simulink model "yaduraj_mli_231040124"  (R2023a)
settings: Solver=ode3  StartTime=0.0  StopTime=.05  RelTol=1e-3  EnableMultiTasking=on
InitFcn:
  | Fs=1550;
  | Ts=1/1550;
libraries: simulink x42, spsIGBTDiodeLib x36, spsDCVoltageSourceLib x9, spsVoltageMeasurementLib x9, spsSeriesRLCBranchLib x3, spsGroundLib x2, sps_lib x1
settings Model: Creator=yadur  LastModifiedBy=yadur
settings SolverCC: AlgebraicLoopSolver=TrustRegion  AutoInsertRateTranBlk=on
settings DataIOCC: SaveFormat=StructureWithTime  ReturnWorkspaceOutputs=off
settings DebuggingCC: ArithmeticOperatorsInVariantConditions=warning
settings SFSimCC: CustomCodeUndefinedFunction=UseInterfaceOnly

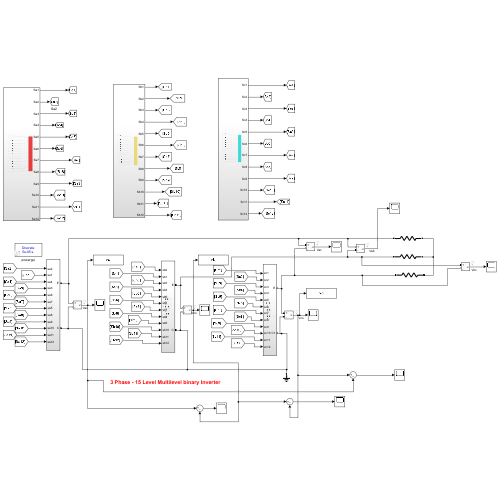
[thumbnail: Simulink's stored preview of the top-level diagram]
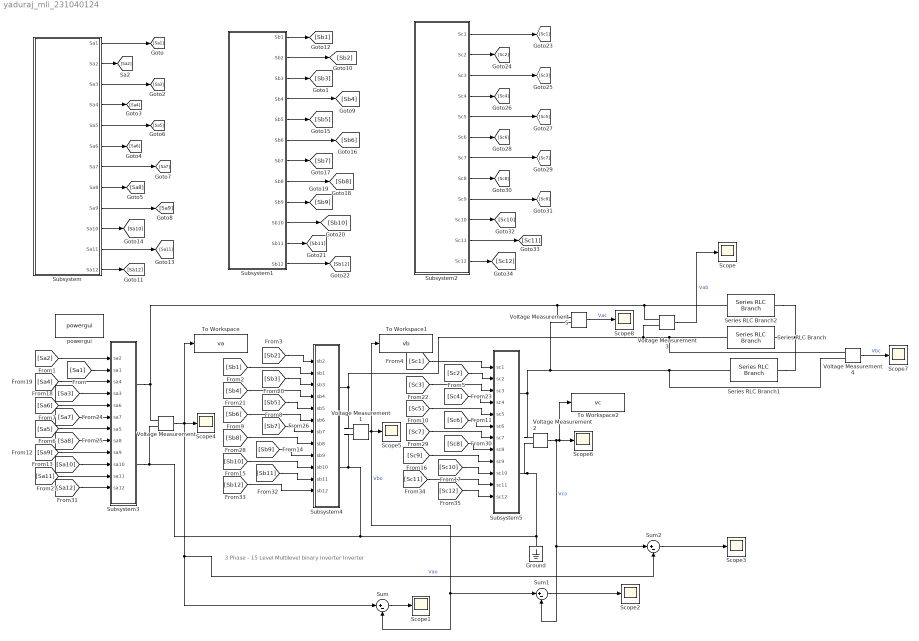
== system yaduraj_mli_231040124 ==
  note: 3 Phase - 15 Level Multilevel binary Inverter Inverter
  Ground : spsGroundLib/Ground  LConnTagsString=a
  Scope{,1..8} (9 alike) : Scope
  Series RLC Branch : spsSeriesRLCBranchLib/Series RLC Branch  LConnTagsString=__new0  RConnTagsString=__new0  BranchType=R  Resistance=1  Inductance=1e-3  SetiL0=off  InitialCurrent=0  Capacitance=1e-6  Setx0=off  InitialVoltage=0  Measurements=None
  Series RLC Branch1 : spsSeriesRLCBranchLib/Series RLC Branch  LConnTagsString=__new0  RConnTagsString=__new0  BranchType=R  Resistance=1  Inductance=1e-3  SetiL0=off  InitialCurrent=0  Capacitance=1e-6  Setx0=off  InitialVoltage=0  Measurements=None
  Series RLC Branch2 : spsSeriesRLCBranchLib/Series RLC Branch  LConnTagsString=__new0  RConnTagsString=__new0  BranchType=R  Resistance=1  Inductance=1e-3  SetiL0=off  InitialCurrent=0  Capacitance=1e-6  Setx0=off  InitialVoltage=0  Measurements=None
  Subsystem : Subsystem
  Subsystem1 : Subsystem
  Subsystem2 : Subsystem
  Subsystem3 : Subsystem
  Subsystem4 : Subsystem
  Subsystem5 : Subsystem
  Sum : Sum  Inputs=|+-
  Sum1 : Sum  Inputs=|+-
  Sum2 : Sum  Inputs=|+-
  To Workspace : ToWorkspace  VariableName=va  SampleTime=-1
      settings: Save2DSignal=2-D array (concatenate along first dimension)
  To Workspace1 : ToWorkspace  VariableName=vb  SampleTime=-1
      settings: Save2DSignal=2-D array (concatenate along first dimension)
  To Workspace2 : ToWorkspace  VariableName=vc  SampleTime=-1
      settings: Save2DSignal=2-D array (concatenate along first dimension)
  Voltage Measurement{,1..5} (6 alike) : spsVoltageMeasurementLib/Voltage Measurement  PhasorSimulation=off  OutputType=Complex  PSBequivalent=0
  powergui : sps_lib/powergui  Priority=1  SimulationMode=Discrete  SampleTime=50e-6  frequency=60  Iterations=50  frequencyindice=0  Pbase=100e6  ErrMax=1e-4  UnitsV=kV  UnitsW=MW  buscounter=0  FunctionMessages=off  echomessages=off  EnableUseOfTLC=off  CurrentSourceSwitches=off  DisableSnubberDevices=off  DisableRonSwitches=off  DisableVfSwitches=off  DisplayEquations=off  AutomaticDiscreteSolvers=off  SolverType=Tustin/Backward Euler (TBE)  Interpol=off  ExternalGateDelay=off  methode=off  Ts=100  x0status=blocks  SPID=on  SwTol=0  HookPort=off  NonlinearTolerance=1e-4  nMaxIteration=100  ContinueOnMaxIteration=off  RestoreLinks=warning  ResistiveCurrentMeasurement=off  Frange=[0:2:500]  Ylog=off  Xlog=on  ShowGrid=off  save=off  variable=ZData  structure=0  ZoomFFT=off  StartTime=0.0  cycles=1  DisplayStyle=1  fundamental=60  FreqAxis=off  MaxFrequency=1000  frequencyindicesteady=1  RmsSteady=1  display=off
  wires:
  Subsystem2/2(Sc2) -> [Sc2]
  Subsystem2/1(Sc1) -> [Sc1]
  Subsystem2/7(Sc7) -> [Sc7]
  Subsystem2/6(Sc6) -> [Sc6]
  Subsystem2/4(Sc4) -> [Sc4]
  Subsystem2/3(Sc3) -> [Sc3]
  Subsystem2/5(Sc5) -> [Sc5]
  [Sc11] -> Subsystem5/11(sc11)
  [Sc6] -> Subsystem5/6(sc6)
  [Sc8] -> Subsystem5/8(sc8)
  [Sc7] -> Subsystem5/7(sc7)
  [Sc10] -> Subsystem5/10(sc10)
  [Sc9] -> Subsystem5/9(sc9)
  Subsystem2/8(Sc8) -> [Sc8]
  [Sc5] -> Subsystem5/5(sc5)
  [Sc4] -> Subsystem5/4(sc4)
  [Sc1] -> Subsystem5/1(sc1)
  Subsystem1/12(Sb12) -> [Sb12]
  Subsystem1/9(Sb9) -> [Sb9]
  [Sc12] -> Subsystem5/12(sc12)
  Subsystem1/6(Sb6) -> [Sb6]
  Subsystem1/11(Sb11) -> [Sb11]
  Subsystem1/5(Sb5) -> [Sb5]
  Subsystem1/8(Sb8) -> [Sb8]
  Subsystem1/7(Sb7) -> [Sb7]
  Subsystem1/2(Sb2) -> [Sb2]
  Subsystem1/4(Sb4) -> [Sb4]
  Subsystem1/3(Sb3) -> [Sb3]
  Subsystem1/1(Sb1) -> [Sb1]
  [Sc2] -> Subsystem5/2(sc2)
  Subsystem/4(Sa4) -> [Sa4]
  Subsystem/10(Sa10) -> [Sa10]
  Subsystem/9(Sa9) -> [Sa9]
  Subsystem/11(Sa11) -> [Sa11]
  [Sa12] -> Subsystem3/12(sa12)
  [Sa9] -> Subsystem3/9(sa9)
  [Sa8] -> Subsystem3/8(sa8)
  [Sa5] -> Subsystem3/7(sa5)
  [Sa6] -> Subsystem3/5(sa6)
  [Sa4] -> Subsystem3/3(sa4)
  [Sa1] -> Subsystem3/2(sa1)
  [Sa2] -> Subsystem3/1(sa2)
  Subsystem/6(Sa6) -> [Sa6]
  [Sa3] -> Subsystem3/4(sa3)
  Subsystem/5(Sa5) -> [Sa5]
  [Sa10] -> Subsystem3/10(sa10)
  Subsystem/1(Sa1) -> [Sa1]
  Subsystem/7(Sa7) -> [Sa7]
  Subsystem1/10(Sb10) -> [Sb10]
  [Sc3] -> Subsystem5/3(sc3)
  Subsystem2/12(Sc12) -> [Sc12]
  Subsystem2/10(Sc10) -> [Sc10]
  Subsystem2/11(Sc11) -> [Sc11]
  [Sa11] -> Subsystem3/11(sa11)
  Subsystem2/9(Sc9) -> [Sc9]
  Subsystem/8(Sa8) -> [Sa8]
  Subsystem/3(Sa3) -> [Sa3]
  Subsystem/12(Sa12) -> [Sa12]
  [Sb12] -> Subsystem4/12(sb12)
  [Sb11] -> Subsystem4/11(sb11)
  [Sb9] -> Subsystem4/9(sb9)
  [Sb10] -> Subsystem4/10(sb10)
  [Sb8] -> Subsystem4/8(sb8)
  Subsystem/2(Sa2) -> [Sa2]
  [Sb7] -> Subsystem4/7(sb7)
  [Sb6] -> Subsystem4/6(sb6)
  [Sb3] -> Subsystem4/3(sb3)
  [Sb2] -> Subsystem4/1(sb2)
  [Sb1] -> Subsystem4/2(sb1)
  [Sa7] -> Subsystem3/6(sa7)
  [Sb5] -> Subsystem4/5(sb5)
  [Sb4] -> Subsystem4/4(sb4)
  Voltage Measurement3/1 -> Scope/1  "Vab"
  Voltage Measurement/1 -> Scope4/1, Sum2/2, Sum/1, To Workspace/1  "Vao"
  Voltage Measurement1/1 -> To Workspace1/1, Scope5/1, Sum1/1, Sum/2  "Vbo"
  Sum/1 -> Scope1/1
  Voltage Measurement2/1 -> Scope6/1, To Workspace2/1, Sum2/1, Sum1/2  "Vco"
  Sum1/1 -> Scope2/1
  Sum2/1 -> Scope3/1
  Voltage Measurement4/1 -> Scope7/1  "Vbc"
  Voltage Measurement5/1 -> Scope8/1  "Vac"
  connections:
  Subsystem5/RConn2 -- Voltage Measurement1/LConn2 -- Subsystem4/RConn2 -- Voltage Measurement/LConn2 -- Subsystem3/RConn2 -- Ground/LConn1 -- Voltage Measurement2/LConn2
  Subsystem4/RConn1 -- Voltage Measurement3/LConn2 -- Voltage Measurement4/LConn1 -- Series RLC Branch/LConn1 -- Voltage Measurement1/LConn1
  Subsystem3/RConn1 -- Voltage Measurement5/LConn1 -- Voltage Measurement3/LConn1 -- Series RLC Branch2/LConn1 -- Voltage Measurement/LConn1
  Subsystem5/RConn1 -- Voltage Measurement5/LConn2 -- Voltage Measurement4/LConn2 -- Series RLC Branch1/LConn1 -- Voltage Measurement2/LConn1
  Series RLC Branch1/RConn1 -- Series RLC Branch2/RConn1 -- Series RLC Branch/RConn1

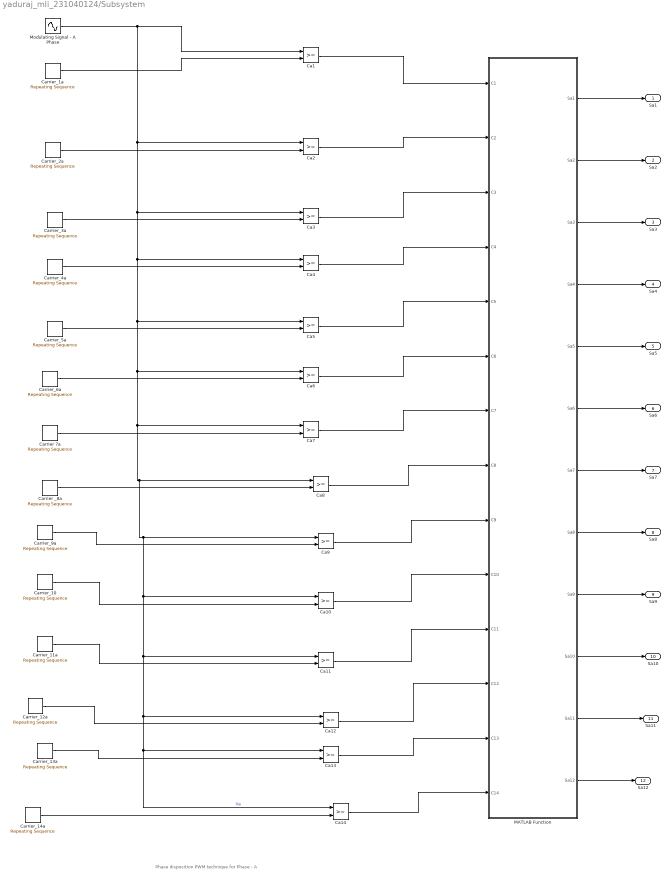
== system yaduraj_mli_231040124/Subsystem ==
  note: Phase disposition PWM technique for Phase - A
  Ca{1..14} (14 alike) : RelationalOperator  OutDataTypeStr=boolean  RndMeth=Simplest  InputSameDT=off
  Carrier 7a : simulink/Sources/Repeating Sequence  rep_seq_t="[0  1/2 1]*Ts"  rep_seq_y="[0 2/14  0]"
  Carrier _8a : simulink/Sources/Repeating Sequence  rep_seq_t="[0  1/2 1]*Ts"  rep_seq_y="[-2/14 0  -2/14  ]"
  Carrier_10 : simulink/Sources/Repeating Sequence  rep_seq_t="[0  1/2 1]*Ts"  rep_seq_y="[-6/14 -4/14  -6/14]"
  Carrier_11a : simulink/Sources/Repeating Sequence  rep_seq_t="[0  1/2 1]*Ts"  rep_seq_y="[-8/14 -6/14  -8/14]"
  Carrier_12a : simulink/Sources/Repeating Sequence  rep_seq_t="[0  1/2 1]*Ts"  rep_seq_y="[-10/14 -8/14  -10/14]"
  Carrier_13a : simulink/Sources/Repeating Sequence  rep_seq_t="[0  1/2 1]*Ts"  rep_seq_y="[-12/14 -10/14  -12/14]"
  Carrier_14a : simulink/Sources/Repeating Sequence  rep_seq_t="[0  1/2 1]*Ts"  rep_seq_y="[-14/14 -12/14  -14/14]"
  Carrier_1a : simulink/Sources/Repeating Sequence  rep_seq_t="[0  1/2 1]*Ts"  rep_seq_y="[12/14 14/14  12/14]"
  Carrier_2a : simulink/Sources/Repeating Sequence  rep_seq_t="[0  1/2 1]*Ts"  rep_seq_y="[10/14 12/14  10/14]"
  Carrier_3a : simulink/Sources/Repeating Sequence  rep_seq_t="[0  1/2 1]*Ts"  rep_seq_y="[8/14 10/14  8/14]"
  Carrier_4a : simulink/Sources/Repeating Sequence  rep_seq_t="[0  1/2 1]*Ts"  rep_seq_y="[6/14 8/14  6/14]"
  Carrier_5a : simulink/Sources/Repeating Sequence  rep_seq_t="[0  1/2 1]*Ts"  rep_seq_y="[4/14 6/14  4/14]"
  Carrier_6a : simulink/Sources/Repeating Sequence  rep_seq_t="[0  1/2 1]*Ts"  rep_seq_y="[2/14 4/14  2/14]"
  Carrier_9a : simulink/Sources/Repeating Sequence  rep_seq_t="[0  1/2 1]*Ts"  rep_seq_y="[-4/14 -2/14  -4/14]"
  MATLAB Function : MATLAB Function  TreatAsAtomicUnit=on
  Modulating Signal - A Phase : Sin  Frequency=2*pi*50  SampleTime=1e-6
  Sa1 : Outport
  Sa2 : Outport  Port=2
  Sa3 : Outport  Port=3
  Sa4 : Outport  Port=4
  Sa5 : Outport  Port=5
  Sa6 : Outport  Port=6
  Sa7 : Outport  Port=7
  Sa8 : Outport  Port=8
  Sa9 : Outport  Port=9
  Sa10 : Outport  Port=10
  Sa11 : Outport  Port=11
  Sa12 : Outport  Port=12
  wires:
  Carrier _8a/1 -> Ca8/2
  Ca8/1 -> MATLAB Function/8(C8)
  Carrier_4a/1 -> Ca4/2
  Ca2/1 -> MATLAB Function/2(C2)
  Carrier_2a/1 -> Ca2/2
  Carrier_9a/1 -> Ca9/2
  Ca3/1 -> MATLAB Function/3(C3)
  MATLAB Function/8(Sa8) -> Sa8/1
  Modulating Signal - A Phase/1 -> Ca14/1, Ca13/1, Ca12/1, Ca11/1, Ca10/1, Ca9/1, Ca8/1, Ca7/1, Ca6/1, Ca5/1, Ca4/1, Ca3/1, Ca2/1, Ca1/1  "Va"
  Carrier_11a/1 -> Ca11/2
  Carrier_3a/1 -> Ca3/2
  Ca5/1 -> MATLAB Function/5(C5)
  MATLAB Function/1(Sa1) -> Sa1/1
  MATLAB Function/4(Sa4) -> Sa4/1
  Carrier_1a/1 -> Ca1/2
  Ca9/1 -> MATLAB Function/9(C9)
  Carrier_5a/1 -> Ca5/2
  MATLAB Function/5(Sa5) -> Sa5/1
  MATLAB Function/9(Sa9) -> Sa9/1
  Ca4/1 -> MATLAB Function/4(C4)
  Ca12/1 -> MATLAB Function/12(C12)
  MATLAB Function/6(Sa6) -> Sa6/1
  Carrier_6a/1 -> Ca6/2
  Ca1/1 -> MATLAB Function/1(C1)
  Ca13/1 -> MATLAB Function/13(C13)
  Ca14/1 -> MATLAB Function/14(C14)
  Ca6/1 -> MATLAB Function/6(C6)
  Carrier_12a/1 -> Ca12/2
  MATLAB Function/3(Sa3) -> Sa3/1
  Carrier_14a/1 -> Ca14/2
  MATLAB Function/10(Sa10) -> Sa10/1
  Ca10/1 -> MATLAB Function/10(C10)
  Carrier 7a/1 -> Ca7/2
  MATLAB Function/12(Sa12) -> Sa12/1
  MATLAB Function/7(Sa7) -> Sa7/1
  Carrier_10/1 -> Ca10/2
  Ca7/1 -> MATLAB Function/7(C7)
  Carrier_13a/1 -> Ca13/2
  MATLAB Function/2(Sa2) -> Sa2/1
  Ca11/1 -> MATLAB Function/11(C11)
  MATLAB Function/11(Sa11) -> Sa11/1

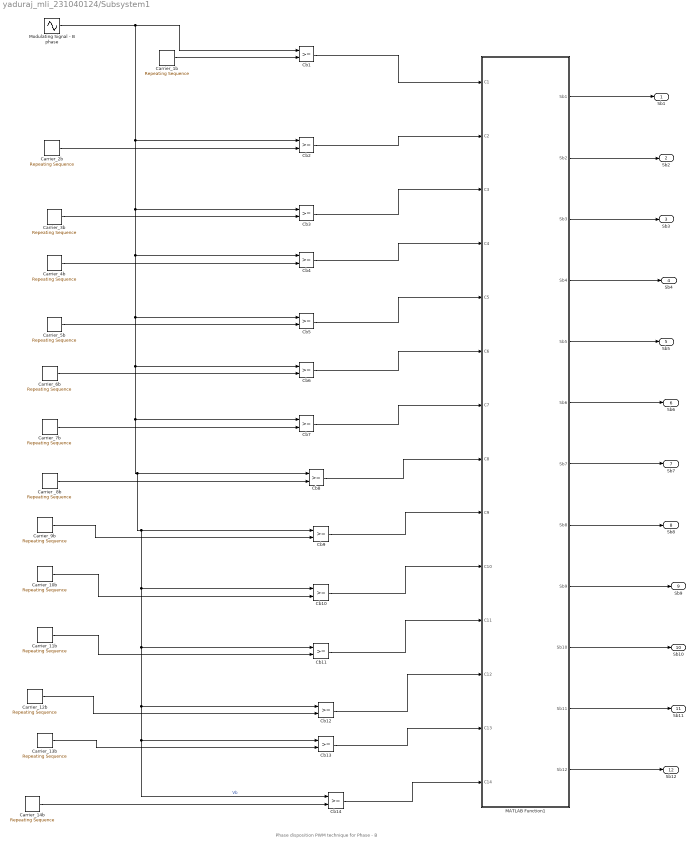
== system yaduraj_mli_231040124/Subsystem1 ==
  note: Phase disposition PWM technique for Phase - B
  Carrier _8b : simulink/Sources/Repeating Sequence  rep_seq_t="[0  1/2 1]*Ts"  rep_seq_y="[-2/14 0  -2/14  ]"
  Carrier_10b : simulink/Sources/Repeating Sequence  rep_seq_t="[0  1/2 1]*Ts"  rep_seq_y="[-6/14 -4/14  -6/14]"
  Carrier_11b : simulink/Sources/Repeating Sequence  rep_seq_t="[0  1/2 1]*Ts"  rep_seq_y="[-8/14 -6/14  -8/14]"
  Carrier_12b : simulink/Sources/Repeating Sequence  rep_seq_t="[0  1/2 1]*Ts"  rep_seq_y="[-10/14 -8/14  -10/14]"
  Carrier_13b : simulink/Sources/Repeating Sequence  rep_seq_t="[0  1/2 1]*Ts"  rep_seq_y="[-12/14 -10/14  -12/14]"
  Carrier_14b : simulink/Sources/Repeating Sequence  rep_seq_t="[0  1/2 1]*Ts"  rep_seq_y="[-14/14 -12/14  -14/14]"
  Carrier_1b : simulink/Sources/Repeating Sequence  rep_seq_t="[0  1/2 1]*Ts"  rep_seq_y="[12/14 14/14  12/14]"
  Carrier_2b : simulink/Sources/Repeating Sequence  rep_seq_t="[0  1/2 1]*Ts"  rep_seq_y="[10/14 12/14  10/14]"
  Carrier_3b : simulink/Sources/Repeating Sequence  rep_seq_t="[0  1/2 1]*Ts"  rep_seq_y="[8/14 10/14  8/14]"
  Carrier_4b : simulink/Sources/Repeating Sequence  rep_seq_t="[0  1/2 1]*Ts"  rep_seq_y="[6/14 8/14  6/14]"
  Carrier_5b : simulink/Sources/Repeating Sequence  rep_seq_t="[0  1/2 1]*Ts"  rep_seq_y="[4/14 6/14  4/14]"
  Carrier_6b : simulink/Sources/Repeating Sequence  rep_seq_t="[0  1/2 1]*Ts"  rep_seq_y="[2/14 4/14  2/14]"
  Carrier_7b : simulink/Sources/Repeating Sequence  rep_seq_t="[0  1/2 1]*Ts"  rep_seq_y="[0 2/14  0]"
  Carrier_9b : simulink/Sources/Repeating Sequence  rep_seq_t="[0  1/2 1]*Ts"  rep_seq_y="[-4/14 -2/14  -4/14]"
  Cb{1..14} (14 alike) : RelationalOperator  OutDataTypeStr=boolean  RndMeth=Simplest  InputSameDT=off
  MATLAB Function1 : MATLAB Function  TreatAsAtomicUnit=on
  Modulating Signal - B phase : Sin  Amplitude=1.01  Frequency=2*pi*50  Phase=-2*pi/3  SampleTime=1e-6  VectorParams1D=off
  Sb1 : Outport
  Sb2 : Outport  Port=2
  Sb3 : Outport  Port=3
  Sb4 : Outport  Port=4
  Sb5 : Outport  Port=5
  Sb6 : Outport  Port=6
  Sb7 : Outport  Port=7
  Sb8 : Outport  Port=8
  Sb9 : Outport  Port=9
  Sb10 : Outport  Port=10
  Sb11 : Outport  Port=11
  Sb12 : Outport  Port=12
  wires:
  Cb2/1 -> MATLAB Function1/2(C2)
  Carrier_4b/1 -> Cb4/2
  Carrier_12b/1 -> Cb12/2
  Carrier_6b/1 -> Cb6/2
  Carrier_11b/1 -> Cb11/2
  Modulating Signal - B phase/1 -> Cb14/1, Cb13/1, Cb12/1, Cb11/1, Cb10/1, Cb9/1, Cb8/1, Cb7/1, Cb6/1, Cb5/1, Cb4/1, Cb3/1, Cb2/1, Cb1/1  "Vb"
  Cb4/1 -> MATLAB Function1/4(C4)
  MATLAB Function1/7(Sb7) -> Sb7/1
  Cb3/1 -> MATLAB Function1/3(C3)
  Carrier_2b/1 -> Cb2/2
  Cb12/1 -> MATLAB Function1/12(C12)
  Carrier_3b/1 -> Cb3/2
  Carrier_13b/1 -> Cb13/2
  Cb8/1 -> MATLAB Function1/8(C8)
  Carrier_7b/1 -> Cb7/2
  Cb1/1 -> MATLAB Function1/1(C1)
  Cb5/1 -> MATLAB Function1/5(C5)
  Carrier _8b/1 -> Cb8/2
  Cb6/1 -> MATLAB Function1/6(C6)
  Carrier_9b/1 -> Cb9/2
  Cb13/1 -> MATLAB Function1/13(C13)
  MATLAB Function1/4(Sb4) -> Sb4/1
  Cb14/1 -> MATLAB Function1/14(C14)
  Cb11/1 -> MATLAB Function1/11(C11)
  MATLAB Function1/6(Sb6) -> Sb6/1
  Carrier_5b/1 -> Cb5/2
  Carrier_10b/1 -> Cb10/2
  MATLAB Function1/9(Sb9) -> Sb9/1
  Cb10/1 -> MATLAB Function1/10(C10)
  Carrier_14b/1 -> Cb14/2
  MATLAB Function1/11(Sb11) -> Sb11/1
  Cb7/1 -> MATLAB Function1/7(C7)
  Carrier_1b/1 -> Cb1/2
  Cb9/1 -> MATLAB Function1/9(C9)
  MATLAB Function1/1(Sb1) -> Sb1/1
  MATLAB Function1/2(Sb2) -> Sb2/1
  MATLAB Function1/10(Sb10) -> Sb10/1
  MATLAB Function1/3(Sb3) -> Sb3/1
  MATLAB Function1/5(Sb5) -> Sb5/1
  MATLAB Function1/12(Sb12) -> Sb12/1
  MATLAB Function1/8(Sb8) -> Sb8/1

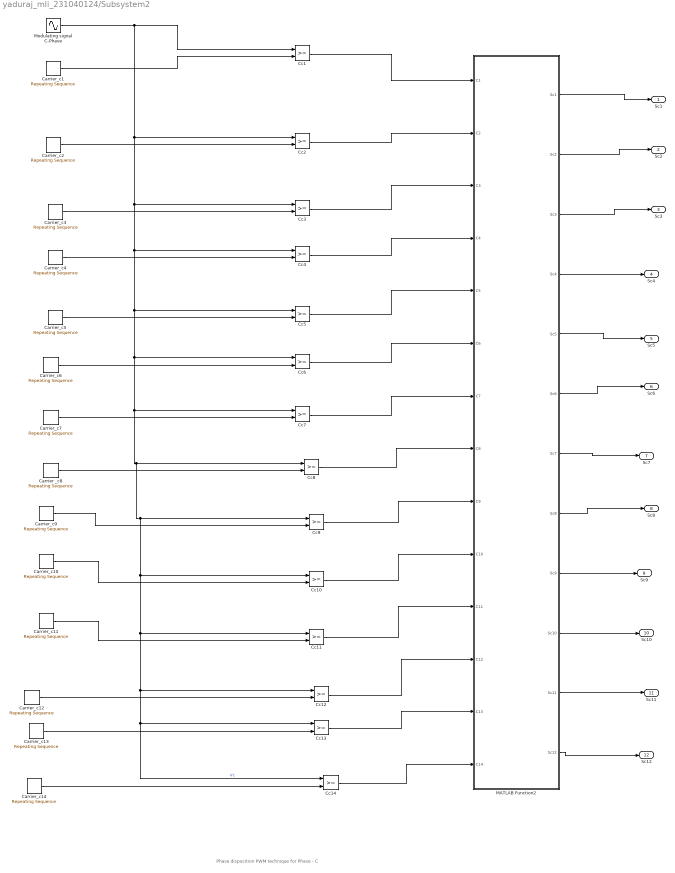
== system yaduraj_mli_231040124/Subsystem2 ==
  note: Phase disposition PWM technique for Phase - C
  Carrier _c8 : simulink/Sources/Repeating Sequence  rep_seq_t="[0  1/2 1]*Ts"  rep_seq_y="[-2/14 0  -2/14  ]"
  Carrier_c1 : simulink/Sources/Repeating Sequence  rep_seq_t="[0  1/2 1]*Ts"  rep_seq_y="[12/14 14/14  12/14]"
  Carrier_c10 : simulink/Sources/Repeating Sequence  rep_seq_t="[0  1/2 1]*Ts"  rep_seq_y="[-6/14 -4/14  -6/14]"
  Carrier_c11 : simulink/Sources/Repeating Sequence  rep_seq_t="[0  1/2 1]*Ts"  rep_seq_y="[-8/14 -6/14  -8/14]"
  Carrier_c12 : simulink/Sources/Repeating Sequence  rep_seq_t="[0  1/2 1]*Ts"  rep_seq_y="[-10/14 -8/14  -10/14]"
  Carrier_c13 : simulink/Sources/Repeating Sequence  rep_seq_t="[0  1/2 1]*Ts"  rep_seq_y="[-12/14 -10/14  -12/14]"
  Carrier_c14 : simulink/Sources/Repeating Sequence  rep_seq_t="[0  1/2 1]*Ts"  rep_seq_y="[-14/14 -12/14  -14/14]"
  Carrier_c2 : simulink/Sources/Repeating Sequence  rep_seq_t="[0  1/2 1]*Ts"  rep_seq_y="[10/14 12/14  10/14]"
  Carrier_c3 : simulink/Sources/Repeating Sequence  rep_seq_t="[0  1/2 1]*Ts"  rep_seq_y="[8/14 10/14  8/14]"
  Carrier_c4 : simulink/Sources/Repeating Sequence  rep_seq_t="[0  1/2 1]*Ts"  rep_seq_y="[6/14 8/14  6/14]"
  Carrier_c5 : simulink/Sources/Repeating Sequence  rep_seq_t="[0  1/2 1]*Ts"  rep_seq_y="[4/14 6/14  4/14]"
  Carrier_c6 : simulink/Sources/Repeating Sequence  rep_seq_t="[0  1/2 1]*Ts"  rep_seq_y="[2/14 4/14  2/14]"
  Carrier_c7 : simulink/Sources/Repeating Sequence  rep_seq_t="[0  1/2 1]*Ts"  rep_seq_y="[0 2/14  0]"
  Carrier_c9 : simulink/Sources/Repeating Sequence  rep_seq_t="[0  1/2 1]*Ts"  rep_seq_y="[-4/14 -2/14  -4/14]"
  Cc{1..14} (14 alike) : RelationalOperator  OutDataTypeStr=boolean  RndMeth=Simplest  InputSameDT=off
  MATLAB Function2 : MATLAB Function  TreatAsAtomicUnit=on
  Modulating signal C-Phase : Sin  Amplitude=1.01  Frequency=2*pi*50  Phase=-4*pi/3  SampleTime=1e-6  VectorParams1D=off
  Sc1 : Outport
  Sc2 : Outport  Port=2
  Sc3 : Outport  Port=3
  Sc4 : Outport  Port=4
  Sc5 : Outport  Port=5
  Sc6 : Outport  Port=6
  Sc7 : Outport  Port=7
  Sc8 : Outport  Port=8
  Sc9 : Outport  Port=9
  Sc10 : Outport  Port=10
  Sc11 : Outport  Port=11
  Sc12 : Outport  Port=12
  wires:
  MATLAB Function2/4(Sc4) -> Sc4/1
  Carrier_c5/1 -> Cc5/2
  Modulating signal C-Phase/1 -> Cc14/1, Cc13/1, Cc12/1, Cc11/1, Cc10/1, Cc9/1, Cc8/1, Cc7/1, Cc6/1, Cc5/1, Cc4/1, Cc3/1, Cc2/1, Cc1/1  "Vc"
  MATLAB Function2/1(Sc1) -> Sc1/1
  Carrier_c12/1 -> Cc12/2
  Cc4/1 -> MATLAB Function2/4(C4)
  MATLAB Function2/12(Sc12) -> Sc12/1
  Cc12/1 -> MATLAB Function2/12(C12)
  MATLAB Function2/9(Sc9) -> Sc9/1
  Cc7/1 -> MATLAB Function2/7(C7)
  Carrier_c13/1 -> Cc13/2
  Carrier_c11/1 -> Cc11/2
  Cc10/1 -> MATLAB Function2/10(C10)
  Carrier_c7/1 -> Cc7/2
  Carrier_c6/1 -> Cc6/2
  Carrier_c3/1 -> Cc3/2
  Carrier _c8/1 -> Cc8/2
  MATLAB Function2/10(Sc10) -> Sc10/1
  Cc5/1 -> MATLAB Function2/5(C5)
  Cc11/1 -> MATLAB Function2/11(C11)
  Carrier_c10/1 -> Cc10/2
  MATLAB Function2/5(Sc5) -> Sc5/1
  Carrier_c2/1 -> Cc2/2
  Cc13/1 -> MATLAB Function2/13(C13)
  Cc8/1 -> MATLAB Function2/8(C8)
  Cc2/1 -> MATLAB Function2/2(C2)
  Cc6/1 -> MATLAB Function2/6(C6)
  Carrier_c9/1 -> Cc9/2
  Carrier_c14/1 -> Cc14/2
  Cc3/1 -> MATLAB Function2/3(C3)
  Carrier_c4/1 -> Cc4/2
  Cc1/1 -> MATLAB Function2/1(C1)
  Cc14/1 -> MATLAB Function2/14(C14)
  Carrier_c1/1 -> Cc1/2
  MATLAB Function2/7(Sc7) -> Sc7/1
  Cc9/1 -> MATLAB Function2/9(C9)
  MATLAB Function2/3(Sc3) -> Sc3/1
  MATLAB Function2/11(Sc11) -> Sc11/1
  MATLAB Function2/6(Sc6) -> Sc6/1
  MATLAB Function2/2(Sc2) -> Sc2/1
  MATLAB Function2/8(Sc8) -> Sc8/1

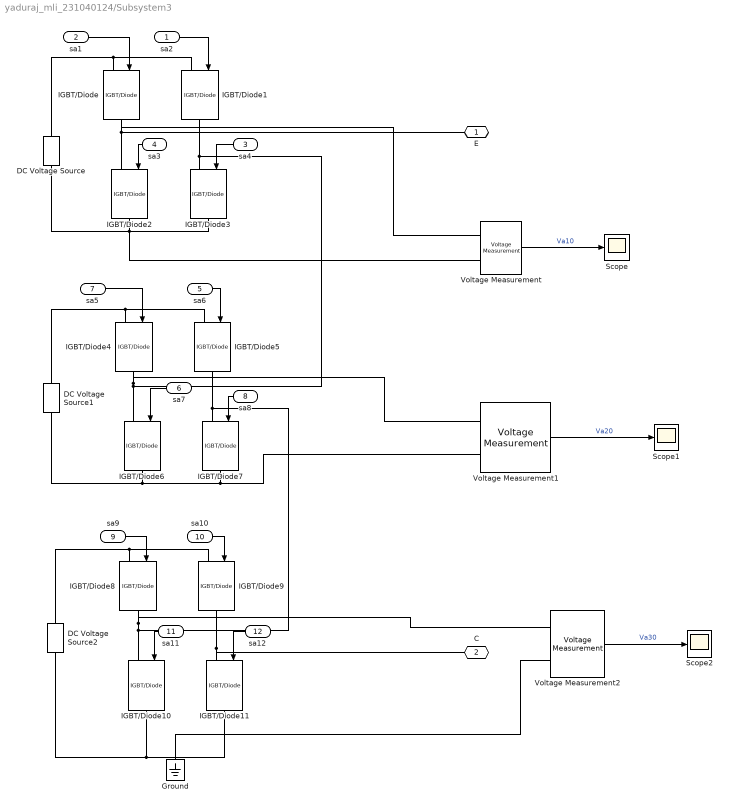
== system yaduraj_mli_231040124/Subsystem3 ==
  sa2 : Inport
  sa1 : Inport  Port=2
  sa4 : Inport  Port=3
  sa3 : Inport  Port=4
  sa6 : Inport  Port=5
  sa7 : Inport  Port=6
  sa5 : Inport  Port=7
  sa8 : Inport  Port=8
  sa9 : Inport  Port=9
  sa10 : Inport  Port=10
  sa11 : Inport  Port=11
  sa12 : Inport  Port=12
  DC Voltage Source : spsDCVoltageSourceLib/DC Voltage Source  Amplitude=100  Measurements=None
  DC Voltage Source1 : spsDCVoltageSourceLib/DC Voltage Source  Amplitude=200  Measurements=None
  DC Voltage Source2 : spsDCVoltageSourceLib/DC Voltage Source  Amplitude=400  Measurements=None
  Ground : spsGroundLib/Ground  LConnTagsString=a
  IGBT/Diode{,1..11} (12 alike) : spsIGBTDiodeLib/IGBT//Diode  Ron=1e-3  Rs=1e5  Cs=inf  Measurements=off
  Scope : Scope
  Scope1 : Scope
  Scope2 : Scope
  Voltage Measurement : spsVoltageMeasurementLib/Voltage Measurement  PhasorSimulation=off  OutputType=Complex  PSBequivalent=0
  Voltage Measurement1 : spsVoltageMeasurementLib/Voltage Measurement  PhasorSimulation=off  OutputType=Complex  PSBequivalent=0
  Voltage Measurement2 : spsVoltageMeasurementLib/Voltage Measurement  PhasorSimulation=off  OutputType=Complex  PSBequivalent=0
  E : PMIOPort  Side=Right
  C : PMIOPort  Port=2  Side=Right
  wires:
  sa5/1 -> IGBT/Diode4/1
  sa3/1 -> IGBT/Diode2/1
  sa10/1 -> IGBT/Diode9/1
  sa8/1 -> IGBT/Diode7/1
  sa1/1 -> IGBT/Diode/1
  sa11/1 -> IGBT/Diode10/1
  sa7/1 -> IGBT/Diode6/1
  sa2/1 -> IGBT/Diode1/1
  sa9/1 -> IGBT/Diode8/1
  sa6/1 -> IGBT/Diode5/1
  sa4/1 -> IGBT/Diode3/1
  sa12/1 -> IGBT/Diode11/1
  Voltage Measurement/1 -> Scope/1  "Va10"
  Voltage Measurement1/1 -> Scope1/1  "Va20"
  Voltage Measurement2/1 -> Scope2/1  "Va30"
  connections:
  IGBT/Diode6/LConn1 -- Voltage Measurement1/LConn1 -- IGBT/Diode4/RConn1 -- IGBT/Diode1/RConn1 -- IGBT/Diode3/LConn1
  IGBT/Diode10/LConn1 -- Voltage Measurement2/LConn1 -- IGBT/Diode8/RConn1 -- IGBT/Diode5/RConn1 -- IGBT/Diode7/LConn1
  DC Voltage Source2/RConn1 -- IGBT/Diode9/LConn1 -- IGBT/Diode8/LConn1
  DC Voltage Source1/RConn1 -- IGBT/Diode5/LConn1 -- IGBT/Diode4/LConn1
  DC Voltage Source/LConn1 -- Voltage Measurement/LConn2 -- IGBT/Diode2/RConn1 -- IGBT/Diode3/RConn1
  IGBT/Diode11/RConn1 -- DC Voltage Source2/LConn1 -- IGBT/Diode10/RConn1
  DC Voltage Source/RConn1 -- IGBT/Diode/LConn1 -- IGBT/Diode1/LConn1
  DC Voltage Source1/LConn1 -- Voltage Measurement1/LConn2 -- IGBT/Diode7/RConn1 -- IGBT/Diode6/RConn1
  IGBT/Diode2/LConn1 -- Voltage Measurement/LConn1 -- E/RConn1 -- IGBT/Diode/RConn1
  IGBT/Diode9/RConn1 -- IGBT/Diode11/LConn1 -- C/RConn1
  Voltage Measurement2/LConn2 -- Ground/LConn1

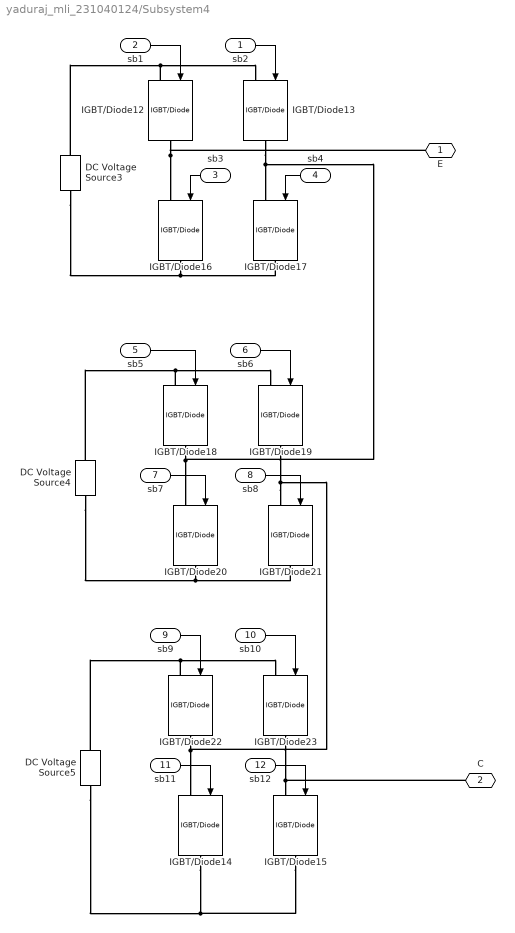
== system yaduraj_mli_231040124/Subsystem4 ==
  sb2 : Inport
  sb1 : Inport  Port=2
  sb3 : Inport  Port=3
  sb4 : Inport  Port=4
  sb5 : Inport  Port=5
  sb6 : Inport  Port=6
  sb7 : Inport  Port=7
  sb8 : Inport  Port=8
  sb9 : Inport  Port=9
  sb10 : Inport  Port=10
  sb11 : Inport  Port=11
  sb12 : Inport  Port=12
  DC Voltage Source3 : spsDCVoltageSourceLib/DC Voltage Source  Amplitude=100  Measurements=None
  DC Voltage Source4 : spsDCVoltageSourceLib/DC Voltage Source  Amplitude=200  Measurements=None
  DC Voltage Source5 : spsDCVoltageSourceLib/DC Voltage Source  Amplitude=400  Measurements=None
  IGBT/Diode{12..23} (12 alike) : spsIGBTDiodeLib/IGBT//Diode  Ron=1e-3  Rs=1e5  Cs=inf  Measurements=off
  E : PMIOPort  Side=Right
  C : PMIOPort  Port=2  Side=Right
  wires:
  sb4/1 -> IGBT/Diode17/1
  sb3/1 -> IGBT/Diode16/1
  sb1/1 -> IGBT/Diode12/1
  sb9/1 -> IGBT/Diode22/1
  sb12/1 -> IGBT/Diode15/1
  sb6/1 -> IGBT/Diode19/1
  sb7/1 -> IGBT/Diode20/1
  sb5/1 -> IGBT/Diode18/1
  sb2/1 -> IGBT/Diode13/1
  sb10/1 -> IGBT/Diode23/1
  sb11/1 -> IGBT/Diode14/1
  sb8/1 -> IGBT/Diode21/1
  connections:
  DC Voltage Source3/RConn1 -- IGBT/Diode13/LConn1 -- IGBT/Diode12/LConn1
  IGBT/Diode23/RConn1 -- IGBT/Diode15/LConn1 -- C/RConn1
  DC Voltage Source5/RConn1 -- IGBT/Diode23/LConn1 -- IGBT/Diode22/LConn1
  DC Voltage Source3/LConn1 -- IGBT/Diode16/RConn1 -- IGBT/Diode17/RConn1
  IGBT/Diode15/RConn1 -- DC Voltage Source5/LConn1 -- IGBT/Diode14/RConn1
  IGBT/Diode21/LConn1 -- IGBT/Diode19/RConn1 -- IGBT/Diode22/RConn1 -- IGBT/Diode14/LConn1
  DC Voltage Source4/RConn1 -- IGBT/Diode19/LConn1 -- IGBT/Diode18/LConn1
  DC Voltage Source4/LConn1 -- IGBT/Diode20/RConn1 -- IGBT/Diode21/RConn1
  IGBT/Diode13/RConn1 -- IGBT/Diode20/LConn1 -- IGBT/Diode18/RConn1 -- IGBT/Diode17/LConn1
  IGBT/Diode12/RConn1 -- E/RConn1 -- IGBT/Diode16/LConn1

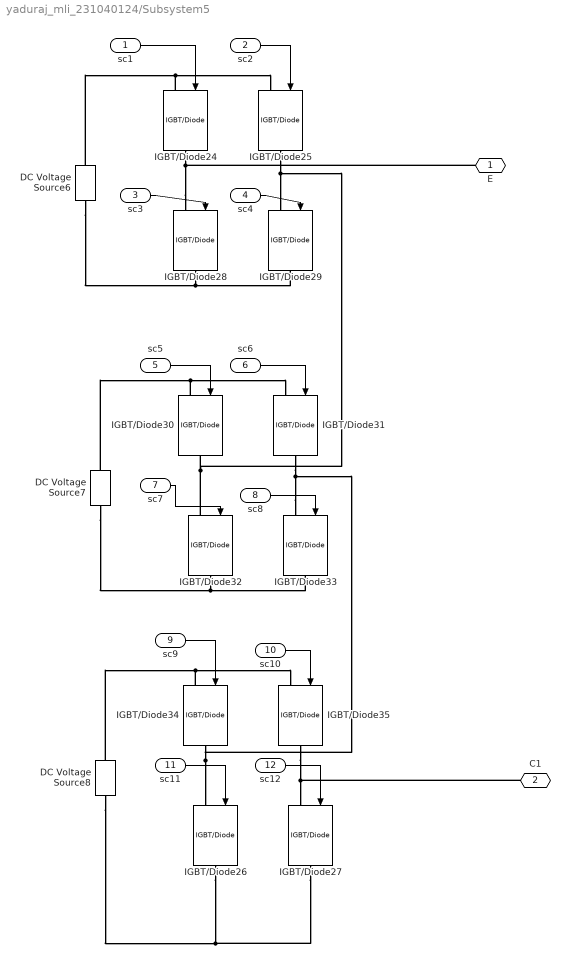
== system yaduraj_mli_231040124/Subsystem5 ==
  sc1 : Inport
  sc2 : Inport  Port=2
  sc3 : Inport  Port=3
  sc4 : Inport  Port=4
  sc5 : Inport  Port=5
  sc6 : Inport  Port=6
  sc7 : Inport  Port=7
  sc8 : Inport  Port=8
  sc9 : Inport  Port=9
  sc10 : Inport  Port=10
  sc11 : Inport  Port=11
  sc12 : Inport  Port=12
  DC Voltage Source6 : spsDCVoltageSourceLib/DC Voltage Source  Amplitude=100  Measurements=None
  DC Voltage Source7 : spsDCVoltageSourceLib/DC Voltage Source  Amplitude=200  Measurements=None
  DC Voltage Source8 : spsDCVoltageSourceLib/DC Voltage Source  Amplitude=400  Measurements=None
  IGBT/Diode{24..35} (12 alike) : spsIGBTDiodeLib/IGBT//Diode  Ron=1e-3  Rs=1e5  Cs=inf  Measurements=off
  E : PMIOPort  Side=Right
  C1 : PMIOPort  Port=2  Side=Right
  wires:
  sc1/1 -> IGBT/Diode24/1
  sc8/1 -> IGBT/Diode33/1
  sc5/1 -> IGBT/Diode30/1
  sc2/1 -> IGBT/Diode25/1
  sc7/1 -> IGBT/Diode32/1
  sc12/1 -> IGBT/Diode27/1
  sc3/1 -> IGBT/Diode28/1
  sc6/1 -> IGBT/Diode31/1
  sc9/1 -> IGBT/Diode34/1
  sc11/1 -> IGBT/Diode26/1
  sc10/1 -> IGBT/Diode35/1
  sc4/1 -> IGBT/Diode29/1
  connections:
  C1/RConn1 -- IGBT/Diode35/RConn1 -- IGBT/Diode27/LConn1
  IGBT/Diode33/LConn1 -- IGBT/Diode31/RConn1 -- IGBT/Diode34/RConn1 -- IGBT/Diode26/LConn1
  IGBT/Diode27/RConn1 -- DC Voltage Source8/LConn1 -- IGBT/Diode26/RConn1
  IGBT/Diode28/LConn1 -- IGBT/Diode24/RConn1 -- E/RConn1
  DC Voltage Source6/RConn1 -- IGBT/Diode25/LConn1 -- IGBT/Diode24/LConn1
  DC Voltage Source7/RConn1 -- IGBT/Diode31/LConn1 -- IGBT/Diode30/LConn1
  DC Voltage Source8/RConn1 -- IGBT/Diode35/LConn1 -- IGBT/Diode34/LConn1
  DC Voltage Source7/LConn1 -- IGBT/Diode32/RConn1 -- IGBT/Diode33/RConn1
  DC Voltage Source6/LConn1 -- IGBT/Diode28/RConn1 -- IGBT/Diode29/RConn1
  IGBT/Diode32/LConn1 -- IGBT/Diode30/RConn1 -- IGBT/Diode29/LConn1 -- IGBT/Diode25/RConn1

== matlab function yaduraj_mli_231040124/Subsystem1/MATLAB Function1 ==
  data: C1 input; Sb1 output; C2 input; C3 input; C4 input; C5 input; C6 input; C7 input; C8 input; C9 input; C10 input; C11 input; C12 input; C13 input; C14 input; Sb2 output; Sb3 output; Sb4 output; Sb5 output; Sb6 output; Sb7 output; Sb8 output; Sb9 output; Sb10 output; Sb11 output; Sb12 output
function [Sb1,Sb2,Sb3,Sb4,Sb5,Sb6,Sb7,Sb8,Sb9,Sb10,Sb11,Sb12] = fcn(C1,C2,C3,C4,C5,C6,C7,C8,C9,C10,C11,C12,C13,C14)

Sb1=0;
Sb2=0;
Sb3=0;
Sb4=0;
Sb5=0;
Sb6=0;
Sb7=0;
Sb8=0;
Sb9=0;
Sb10=0;
Sb11=0;
Sb12=0;


spwm_sum=C1+C2+C3+C4+C5+C6+C7+C8+C9+C10+C11+C12+C13+C14;

if(spwm_sum==14)     % V_out=7Vdc

Sb1=1;
Sb2=0;
Sb3=0;
Sb4=1;
Sb5=1;
Sb6=0;
Sb7=0;
Sb8=1;
Sb9=1;
Sb10=0;
Sb11=0;
Sb12=1;

elseif (spwm_sum==13)


    % V_out=6Vdc

 Sb1=1;
Sb2=1;
Sb3=0;
Sb4=0;
Sb5=1;
Sb6=0;
Sb7=0;
Sb8=1;
Sb9=1;
Sb10=0;
Sb11=0;
Sb12=1;

elseif (spwm_sum==12)

         % V_out=5Vdc

 Sb1=0;
Sb2=1;
Sb3=1;
Sb4=0;
Sb5=1;
Sb6=0;
Sb7=0;
Sb8=1;
Sb9=1;
Sb10=0;
Sb11=0;
Sb12=1;

elseif (spwm_sum==11)
    % V_out=4Vdc

 Sb1=0;
Sb2=0;
Sb3=1;
Sb4=1;
Sb5=1;
Sb6=1;
Sb7=0;
Sb8=0;
Sb9=1;
Sb10=0;
Sb11=0;
Sb12=1;

elseif (spwm_sum==10)

      % V_out=3Vdc

 Sb1=0;
Sb2=1;
Sb3=1;
Sb4=0;
Sb5=1;
Sb6=1;
Sb7=0;
Sb8=0;
Sb9=1;
Sb10=0;
Sb11=0;
Sb12=12;

elseif (spwm_sum==9)


        % V_out=2Vdc

 Sb1=0;
Sb2=0;
Sb3=1;
Sb4=1;
Sb5=0;
Sb6=1;
Sb7=1;
Sb8=0;
Sb9=1;
Sb10=0;
Sb11=0;
Sb12=12;

elseif (spwm_sum==8)


      % V_out=Vdc

 Sb1=0;
Sb2=1;
Sb3=1;
Sb4=0;
Sb5=0;
Sb6=1;
Sb7=1;
Sb8=0;
Sb9=1;
Sb10=0;
Sb11=0;
Sb12=12;

elseif (spwm_sum==7)


   % V_out=0

 Sb1=0;
Sb2=0;
Sb3=1;
Sb4=1;
Sb5=0;
Sb6=0;
Sb7=1;
Sb8=1;
Sb9=1;
Sb10=1;
Sb11=0;
Sb12=0;

elseif (spwm_sum==6)

    % V_out=-Vdc

 Sb1=0;
Sb2=1;
Sb3=1;
Sb4=0;
Sb5=0;
Sb6=0;
Sb7=1;
Sb8=1;
Sb9=1;
Sb10=1;
Sb11=0;
Sb12=0;

elseif (spwm_sum==5)


    % V_out=-2Vdc

 Sb1=0;
Sb2=0;
Sb3=1;
Sb4=1;
Sb5=0;
Sb6=1;
Sb7=1;
Sb8=0;
Sb9=1;
Sb10=1;
Sb11=0;
Sb12=0;

elseif (spwm_sum==4)

        % V_out=-3Vdc

 Sb1=0;
Sb2=1;
Sb3=1;
Sb4=0;
Sb5=0;
Sb6=1;
Sb7=1;
Sb8=0;
Sb9=1;
Sb10=1;
Sb11=0;
Sb12=0;

elseif (spwm_sum==3)

       % V_out=-4Vdc

 Sb1=0;
Sb2=0;
Sb3=1;
Sb4=1;
Sb5=0;
Sb6=0;
Sb7=1;
Sb8=1;
Sb9=0;
Sb10=1;
Sb11=1;
Sb12=0;

elseif (spwm_sum==2)

     % V_out=-5Vdc

 Sb1=0;
Sb2=1;
Sb3=1;
Sb4=0;
Sb5=0;
Sb6=0;
Sb7=1;
Sb8=1;
Sb9=0;
Sb10=1;
Sb11=1;
Sb12=0;

elseif (spwm_sum==1)

    % V_out=-6Vdc

 Sb1=0;
Sb2=0;
Sb3=1;
Sb4=1;
Sb5=0;
Sb6=1;
Sb7=1;
Sb8=0;
Sb9=0;
Sb10=1;
Sb11=1;
Sb12=0;

elseif (spwm_sum==0)


      % V_out=-7Vdc

 Sb1=0;
Sb2=1;
Sb3=1;
Sb4=0;
Sb5=0;
Sb6=1;
Sb7=1;
Sb8=0;
Sb9=0;
Sb10=1;
Sb11=1;
Sb12=0;

end
end

== matlab function yaduraj_mli_231040124/Subsystem/MATLAB Function ==
  data: C1 input; Sa1 output; C2 input; C3 input; C4 input; C5 input; C6 input; C7 input; C8 input; C9 input; C10 input; C11 input; C12 input; C13 input; C14 input; Sa2 output; Sa3 output; Sa4 output; Sa5 output; Sa6 output; Sa7 output; Sa8 output; Sa9 output; Sa10 output; Sa11 output; Sa12 output
function [Sa1,Sa2,Sa3,Sa4,Sa5,Sa6,Sa7,Sa8,Sa9,Sa10,Sa11,Sa12] = fcn(C1,C2,C3,C4,C5,C6,C7,C8,C9,C10,C11,C12,C13,C14)

Sa1=0;
Sa2=0;
Sa3=0;
Sa4=0;
Sa5=0;
Sa6=0;
Sa7=0;
Sa8=0;
Sa9=0;
Sa10=0;
Sa11=0;
Sa12=0;


spwm_sum=C1+C2+C3+C4+C5+C6+C7+C8+C9+C10+C11+C12+C13+C14;

if(spwm_sum==14)     % V_out=7Vdc

Sa1=1;
Sa2=0;
Sa3=0;
Sa4=1;
Sa5=1;
Sa6=0;
Sa7=0;
Sa8=1;
Sa9=1;
Sa10=0;
Sa11=0;
Sa12=1;

elseif (spwm_sum==13)


    % V_out=6Vdc

 Sa1=1;
Sa2=1;
Sa3=0;
Sa4=0;
Sa5=1;
Sa6=0;
Sa7=0;
Sa8=1;
Sa9=1;
Sa10=0;
Sa11=0;
Sa12=1;

elseif (spwm_sum==12)

         % V_out=5Vdc

 Sa1=0;
Sa2=1;
Sa3=1;
Sa4=0;
Sa5=1;
Sa6=0;
Sa7=0;
Sa8=1;
Sa9=1;
Sa10=0;
Sa11=0;
Sa12=1;

elseif (spwm_sum==11)
    % V_out=4Vdc

 Sa1=0;
Sa2=0;
Sa3=1;
Sa4=1;
Sa5=1;
Sa6=1;
Sa7=0;
Sa8=0;
Sa9=1;
Sa10=0;
Sa11=0;
Sa12=1;

elseif (spwm_sum==10)

      % V_out=3Vdc

 Sa1=0;
Sa2=1;
Sa3=1;
Sa4=0;
Sa5=1;
Sa6=1;
Sa7=0;
Sa8=0;
Sa9=1;
Sa10=0;
Sa11=0;
Sa12=12;

elseif (spwm_sum==9)


        % V_out=2Vdc

 Sa1=0;
Sa2=0;
Sa3=1;
Sa4=1;
Sa5=0;
Sa6=1;
Sa7=1;
Sa8=0;
Sa9=1;
Sa10=0;
Sa11=0;
Sa12=12;

elseif (spwm_sum==8)


      % V_out=Vdc

 Sa1=0;
Sa2=1;
Sa3=1;
Sa4=0;
Sa5=0;
Sa6=1;
Sa7=1;
Sa8=0;
Sa9=1;
Sa10=0;
Sa11=0;
Sa12=12;

elseif (spwm_sum==7)


   % V_out=0

 Sa1=0;
Sa2=0;
Sa3=1;
Sa4=1;
Sa5=0;
Sa6=0;
Sa7=1;
Sa8=1;
Sa9=1;
Sa10=1;
Sa11=0;
Sa12=0;

elseif (spwm_sum==6)

    % V_out=-Vdc

 Sa1=0;
Sa2=1;
Sa3=1;
Sa4=0;
Sa5=0;
Sa6=0;
Sa7=1;
Sa8=1;
Sa9=1;
Sa10=1;
Sa11=0;
Sa12=0;

elseif (spwm_sum==5)


    % V_out=-2Vdc

 Sa1=0;
Sa2=0;
Sa3=1;
Sa4=1;
Sa5=0;
Sa6=1;
Sa7=1;
Sa8=0;
Sa9=1;
Sa10=1;
Sa11=0;
Sa12=0;

elseif (spwm_sum==4)

        % V_out=-3Vdc

 Sa1=0;
Sa2=1;
Sa3=1;
Sa4=0;
Sa5=0;
Sa6=1;
Sa7=1;
Sa8=0;
Sa9=1;
Sa10=1;
Sa11=0;
Sa12=0;

elseif (spwm_sum==3)

       % V_out=-4Vdc

 Sa1=0;
Sa2=0;
Sa3=1;
Sa4=1;
Sa5=0;
Sa6=0;
Sa7=1;
Sa8=1;
Sa9=0;
Sa10=1;
Sa11=1;
Sa12=0;

elseif (spwm_sum==2)

     % V_out=-5Vdc

 Sa1=0;
Sa2=1;
Sa3=1;
Sa4=0;
Sa5=0;
Sa6=0;
Sa7=1;
Sa8=1;
Sa9=0;
Sa10=1;
Sa11=1;
Sa12=0;

elseif (spwm_sum==1)

    % V_out=-6Vdc

 Sa1=0;
Sa2=0;
Sa3=1;
Sa4=1;
Sa5=0;
Sa6=1;
Sa7=1;
Sa8=0;
Sa9=0;
Sa10=1;
Sa11=1;
Sa12=0;

elseif (spwm_sum==0)


      % V_out=-7Vdc

 Sa1=0;
Sa2=1;
Sa3=1;
Sa4=0;
Sa5=0;
Sa6=1;
Sa7=1;
Sa8=0;
Sa9=0;
Sa10=1;
Sa11=1;
Sa12=0;

end
end

== matlab function yaduraj_mli_231040124/Subsystem2/MATLAB Function2 ==
  data: C1 input; Sc1 output; C2 input; C3 input; C4 input; C5 input; C6 input; C7 input; C8 input; C9 input; C10 input; C11 input; C12 input; C13 input; C14 input; Sc2 output; Sc3 output; Sc4 output; Sc5 output; Sc6 output; Sc7 output; Sc8 output; Sc9 output; Sc10 output; Sc11 output; Sc12 output
function [Sc1,Sc2,Sc3,Sc4,Sc5,Sc6,Sc7,Sc8,Sc9,Sc10,Sc11,Sc12] = fcn(C1,C2,C3,C4,C5,C6,C7,C8,C9,C10,C11,C12,C13,C14)

Sc1=0;
Sc2=0;
Sc3=0;
Sc4=0;
Sc5=0;
Sc6=0;
Sc7=0;
Sc8=0;
Sc9=0;
Sc10=0;
Sc11=0;
Sc12=0;


spwm_sum=C1+C2+C3+C4+C5+C6+C7+C8+C9+C10+C11+C12+C13+C14;

if(spwm_sum==14)     % V_out=7Vdc

Sc1=1;
Sc2=0;
Sc3=0;
Sc4=1;
Sc5=1;
Sc6=0;
Sc7=0;
Sc8=1;
Sc9=1;
Sc10=0;
Sc11=0;
Sc12=1;

elseif (spwm_sum==13)


    % V_out=6Vdc

 Sc1=1;
Sc2=1;
Sc3=0;
Sc4=0;
Sc5=1;
Sc6=0;
Sc7=0;
Sc8=1;
Sc9=1;
Sc10=0;
Sc11=0;
Sc12=1;

elseif (spwm_sum==12)

         % V_out=5Vdc

 Sc1=0;
Sc2=1;
Sc3=1;
Sc4=0;
Sc5=1;
Sc6=0;
Sc7=0;
Sc8=1;
Sc9=1;
Sc10=0;
Sc11=0;
Sc12=1;

elseif (spwm_sum==11)
    % V_out=4Vdc

 Sc1=0;
Sc2=0;
Sc3=1;
Sc4=1;
Sc5=1;
Sc6=1;
Sc7=0;
Sc8=0;
Sc9=1;
Sc10=0;
Sc11=0;
Sc12=1;

elseif (spwm_sum==10)

      % V_out=3Vdc

 Sc1=0;
Sc2=1;
Sc3=1;
Sc4=0;
Sc5=1;
Sc6=1;
Sc7=0;
Sc8=0;
Sc9=1;
Sc10=0;
Sc11=0;
Sc12=12;

elseif (spwm_sum==9)


        % V_out=2Vdc

 Sc1=0;
Sc2=0;
Sc3=1;
Sc4=1;
Sc5=0;
Sc6=1;
Sc7=1;
Sc8=0;
Sc9=1;
Sc10=0;
Sc11=0;
Sc12=12;

elseif (spwm_sum==8)


      % V_out=Vdc

 Sc1=0;
Sc2=1;
Sc3=1;
Sc4=0;
Sc5=0;
Sc6=1;
Sc7=1;
Sc8=0;
Sc9=1;
Sc10=0;
Sc11=0;
Sc12=12;

elseif (spwm_sum==7)


   % V_out=0

 Sc1=0;
Sc2=0;
Sc3=1;
Sc4=1;
Sc5=0;
Sc6=0;
Sc7=1;
Sc8=1;
Sc9=1;
Sc10=1;
Sc11=0;
Sc12=0;

elseif (spwm_sum==6)

    % V_out=-Vdc

 Sc1=0;
Sc2=1;
Sc3=1;
Sc4=0;
Sc5=0;
Sc6=0;
Sc7=1;
Sc8=1;
Sc9=1;
Sc10=1;
Sc11=0;
Sc12=0;

elseif (spwm_sum==5)


    % V_out=-2Vdc

 Sc1=0;
Sc2=0;
Sc3=1;
Sc4=1;
Sc5=0;
Sc6=1;
Sc7=1;
Sc8=0;
Sc9=1;
Sc10=1;
Sc11=0;
Sc12=0;

elseif (spwm_sum==4)

        % V_out=-3Vdc

 Sc1=0;
Sc2=1;
Sc3=1;
Sc4=0;
Sc5=0;
Sc6=1;
Sc7=1;
Sc8=0;
Sc9=1;
Sc10=1;
Sc11=0;
Sc12=0;

elseif (spwm_sum==3)

       % V_out=-4Vdc

 Sc1=0;
Sc2=0;
Sc3=1;
Sc4=1;
Sc5=0;
Sc6=0;
Sc7=1;
Sc8=1;
Sc9=0;
Sc10=1;
Sc11=1;
Sc12=0;

elseif (spwm_sum==2)

     % V_out=-5Vdc

 Sc1=0;
Sc2=1;
Sc3=1;
Sc4=0;
Sc5=0;
Sc6=0;
Sc7=1;
Sc8=1;
Sc9=0;
Sc10=1;
Sc11=1;
Sc12=0;

elseif (spwm_sum==1)

    % V_out=-6Vdc

 Sc1=0;
Sc2=0;
Sc3=1;
Sc4=1;
Sc5=0;
Sc6=1;
Sc7=1;
Sc8=0;
Sc9=0;
Sc10=1;
Sc11=1;
Sc12=0;

elseif (spwm_sum==0)


      % V_out=-7Vdc

 Sc1=0;
Sc2=1;
Sc3=1;
Sc4=0;
Sc5=0;
Sc6=1;
Sc7=1;
Sc8=0;
Sc9=0;
Sc10=1;
Sc11=1;
Sc12=0;

end
end
